simulink model "MATE_SynchronousMachine"  (R2024b)
settings: Solver=FixedStepDiscrete  StartTime=0.0  StopTime=6  FixedStep=Ts  RelTol=1e-4  EnableMultiTasking=on
PostLoadFcn:
  | Ts=25e-6;offset=4;
InitFcn:
  | Ts=25e-6;offset=4;
undefined symbols (not defined in the file): DiscIntNeverNeededParam, MATE, Phase, Rsnu, Single
libraries: fl_lib x79, nesl_utility x53, ee_lib x16, simetran x5, powerlib_extras x3, simulink_extras x2, simulink x2
(part 1 of 5)
settings Model: ARTEMISmethode_block_infos=$$__separator__$$  Creator=by2815  LastModifiedBy=CD8435
settings SolverCC: AlgebraicLoopSolver=TrustRegion
settings DataIOCC: SaveFormat=Structure  SignalLoggingSaveFormat=ModelDataLogs  SaveOutput=off  SignalLogging=off  SaveTime=off  ReturnWorkspaceOutputs=off  SignalLoggingName=sigsOut
settings OptimizationCC: ExpressionDepthLimit=2147483647  InitFltsAndDblsToZero=on  LifeSpan=inf
settings DebuggingCC: SaveWithParameterizedLinksMsg=none  UnderspecifiedInitializationDetection=Classic  MergeDetectMultiDrivingBlocksExec=none  SignalResolutionControl=TryResolveAllWithWarning  MultiTaskDSMMsg=warning  MultiTaskCondExecSysMsg=none  FcnCallInpInsideContextMsg=warning  AllowSymbolicDim=off  StateNameClashWarn=warning  NonBusSignalsTreatedAsBus=error  SFUnexpectedBacktrackingDiag=warning  SFNoUnconditionalDefaultTransitionDiag=warning  SFExecutionAtInitializationDiag=none  ArithmeticOperatorsInVariantConditions=warning
settings HardwareCC: ProdBitPerPointer=32  ProdBitPerSizeT=32  ProdBitPerPtrDiffT=32  ProdLargestAtomicFloat=None  ProdIntDivRoundTo=Undefined  ProdEndianess=Unspecified  ProdWordSize=32  ProdHWDeviceType=32-bit Generic  TargetUnknown=on
settings ModelReferenceCC: EnableRefExpFcnMdlSchedulingChecks=on  PropagateSignalLabelsOutOfModel=off
settings SFSimCC: SimUseLocalCustomCode=off  CustomCodeUndefinedFunction=UseInterfaceOnly
settings RTWCC: RTWUseLocalCustomCode=off  GPUComputeCapability=3.5
settings CodeAppCC: StateflowObjectComments=on
settings GRTTargetCC: TargetFcnLib=ansi_tfl_tmw.mat  TargetLangStandard=C89/C90 (ANSI)  CombineOutputUpdateFcns=off  GRTInterface=on
settings ConfigComp: CovMetricSettings=dw  CovSaveCumulativeToWorkspaceVar=on  CovSaveSingleToWorkspaceVar=on  CovExternalEMLEnable=off
settings SimscapeCC: SimscapeNormalizeSystem=off

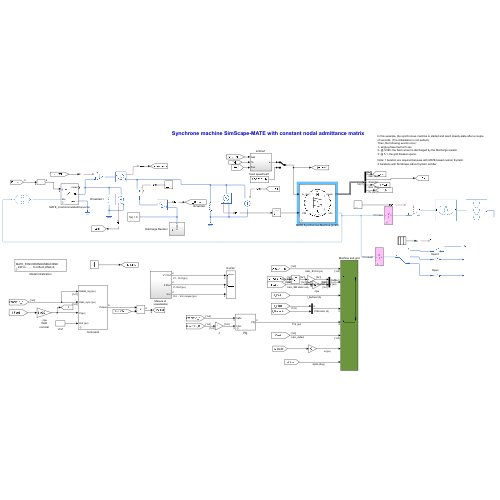
[thumbnail: Simulink's stored preview of the top-level diagram]
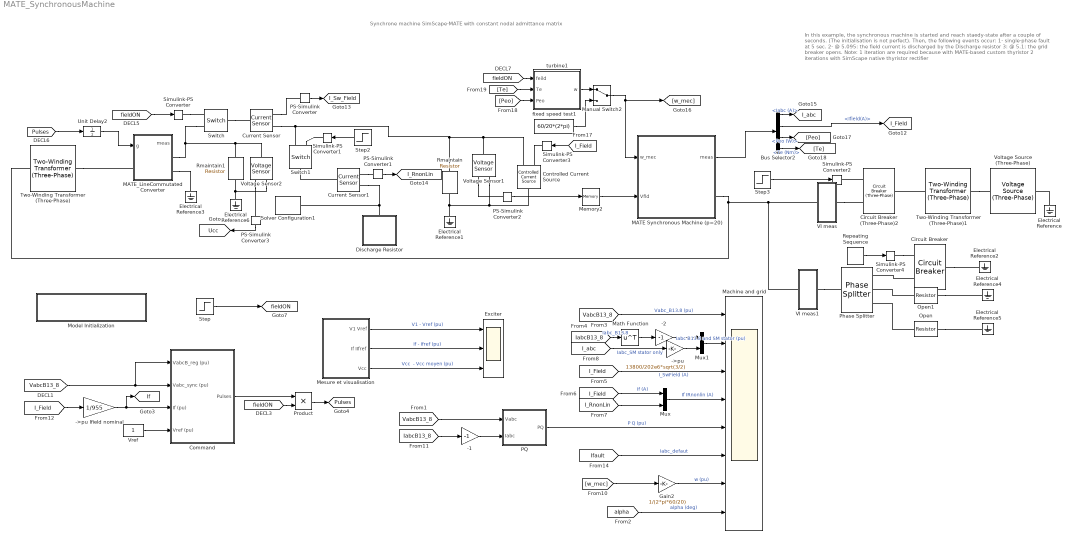
== system MATE_SynchronousMachine ==
  note: In this example, the synchronous machine is started and reach staedy-state after a couple of seconds. (The initialisation is not perfect).
      | Then, the following events occur:
      | 1- single-phase fault at 5 sec.
      | 2- @ 5.095: the field current is discharged by the Discharge resistor
      | 3: @ 5.1: the grid breaker opens.
      |
      | Note: 1 iteration are required because with MATE-based custom thyristor
      | 2 iterations with SimScape native thyristor rectifier
  note: Synchrone machine SimScape-MATE with constant nodal admittance matrix
  -1 : Gain  Gain=-1
  -2 : Gain  Gain=-1
  ->pu : Gain  Gain=13800/202e6*sqrt(3/2)
  ->pu Ifield nominal : Gain  Gain=1/955
  Bus Selector2 : BusSelector  OutputSignals=Iabc (A),Ifield(A),Peo (W),Te (Nm)
  Circuit Breaker : ee_lib/Switches & Breakers/Circuit Breaker  R_closed=0.01 Ohm  G_open=1e-6 1/Ohm  threshold=0.5 V  breaker_behavior=ee.enum.switches.breakerBehavior.zeroCrossingEnable
      settings: InternalSimscapePortConfiguration="{\"Bottom\":[],\"Left\":[{\"id\":\"vT\",\"label\":\"vT\",\"type\":\"input\"},{\"id\":\"p1\",\"label\":\"\",\"type\":\"foundation.electrical.electrical\"}],\"Right\":[{\"id\":\"p2\",\"label\":\"\",\"type\":\"foundation.electrical.electrical\"}],\"Top\":[]}"
  Circuit Breaker (Three-Phase)2 : ee_lib/Switches & Breakers/Circuit Breaker (Three-Phase)  R_closed=0.01 Ohm  G_open=1e-6 1/Ohm  threshold=0.5 V  breaker_behavior=ee.enum.switches.breakerBehavior.zeroCrossingEnable
      settings: InternalSimscapePortConfiguration="{\"Bottom\":[],\"Left\":[{\"id\":\"vT\",\"label\":\"vT\",\"type\":\"input\"},{\"id\":\"N1\",\"label\":\"~1\",\"type\":\"foundation.electrical.three_phase\"}],\"Right\":[{\"id\":\"N2\",\"label\":\"~2\",\"type\":\"foundation.electrical.three_phase\"}],\"Top\":[]}"
  Command : Subsystem  mask{ModOp=Automatique (regulation de tension), Vref=1.0, Iref_man=1.0, K_V=[ 20 300  ], K_I=[ 400  1000 ], Ts=Ts}
      mask prompts: ModOp "Mode d'operation"; Vref "Consigne de tension (pu)"; Iref_man "Consigne de courant (pu)"; K_V "Gain du regulateur de tension [ Kp  Ki ]"; K_I "Gain du regulateur de courant: [ Kp  Ki ]"; Ts "Pas de calcul"
      mask init:
      | Kp_V=K_V(1); Ki_V=K_V(2);
      | Kp_I=K_I(1); Ki_I=K_I(2);
      | if ModOp==1
      |     Auto=1;
      | else
      |     Auto=0;
      | end
      mask TypeOptions ModOp: Automatique (regulation de tension) | Manuel (regulation de courant)
  Controlled Current Source : fl_lib/Electrical/Electrical Sources/Controlled Current Source
  Current Sensor : fl_lib/Electrical/Electrical Sensors/Current Sensor
  Current Sensor1 : fl_lib/Electrical/Electrical Sensors/Current Sensor
  Discharge Resistor : Subsystem
  Electrical Reference{,1..6} (7 alike) : fl_lib/Electrical/Electrical Elements/Electrical Reference
  Exciter : Scope  NumInputPorts=3
  Gain2 : Gain  Gain=1/(2*pi*60/20)
  MATE Synchronous Machine (p=20) : Subsystem  mask(MATE Synchronous Machine (Fixed Admittance)){NominalParameters=[ 202e6  13800   60   955 ], Rtype=Salient (5ft order model), Stator=[ 2.9069E-03  3.0892E-04  3.2164E-03 9.7153E-04 0.0], Field=[ 5.9013E-04*0.128/0.08381   3.0712E-04], Dampers1=[ 1.1900E-02  4.9076E-04   2.0081E-02  1.0365E-03  2.0081E-02  1.0365E-03], PolePairs=20, InitialConditions=-95, InitCurrents=[ 1180 9560 9560 9650 [0 -120 120]-95], Ts=Ts, Parameter19=|, sat=off, DiffSat=off, SatVt=[0 0.7 1 1.4], SatIfd=[0 0.5 1 2], plotsat=off, R0=500, X0=0.11643, nsnf_readonly=0.083912, Parameter18=|}
      mask Parameter19=|
      | Saturation: Saturation is used if selected
      |
      | Open stator saturation curve: field current data in per unit of nominal field current
      | Open stator saturation curve: phase-phase RMS terminal voltage in per unit of nominal voltage
      | Plot saturation curves
      | Zero sequence machine reactance (Ohms): grounding impedance internally connected to the stator Y neutral.
      | Neutral grounding resistance (Ohms): grounding resistance (in series with the impedance) internally connected to the stator Y neutral.
      mask Parameter18=|
      | The stator-to-field coil winding turn ratio (Ns_to_Nf) is found using the following formula:
      |
      | Ns_on_Nf=Lmd*I_fn*(2*pi*f_base)/Vbase
      | where Lmd (d-axis mutual inductance), I_fn (nominal field current), f_base (nominal electric frequency) and Vbase (open-stator machine nominal line-line RMS voltage).
      mask prompts: NominalParameters "Nominal power, voltage, frequency, field current  [ Pn(VA) Vn(Vrms) fn(Hz) ifn(A) ]:"; Rtype "Rotor type"; Stator "Stator  [ Rs(ohm), Ll, Lmd, Lmq(H), Lcanay(H) ]:"; Field "Field  [ Rf'(ohm)  Llfd'(H) ]:"; Dampers1 "Dampers   [ Rkd',Llkd'  Rkq1',Llkq1'  Rkq2' Llkq2' ] (R=ohm,L=H): (Rk2 Lfk2 values not used for salient type machine)"; PolePairs "Pole pairs:"; InitialConditions "Initial rotor angle (deg):"; InitCurrents "Initial currents  Ifd (A) Ia Ib Ic (A) (amplitude)  Ia Ib Ic (deg)(angle )"; Ts "Sample Time (s)"; Parameter19 "text1"; sat "Saturation"; DiffSat "Differential saturation (not available)"; SatVt "Open stator saturation curve: phase-phase RMS voltage (pu of nominal voltage)"; SatIfd "Open stator saturation curve: field current (pu of nominal field current)"; plotsat "Plot saturation curves"; R0 "Neutral grounding resistance (Ohms)"; X0 "Zero sequence machine reactance (Ohms)"; nsnf_readonly "Computed Stator/Field turn ratio (read-only)"; Parameter18 "text2"
      mask help:
      | Implements a 3-phase synchronous machine modelled in the dq rotor reference frame for use with SimScape
      | The model uses a fixed admittance matrix method and is well designed for real-time simulation.
      |
      | The model is 6th order for the round rotor type and 5th order for the salient rotor type (Rk2 Llk2 are internally set to inf in this case).Stator windings are connected in wye to an internal neutral point to which an internal impedance to ground can be selected by the user.
      | If selected, saturation occured in both d- and q- axis, using total flux, for the round and salient rotor type.
      |
      |
      | Parameters: (all values are in SI units)
      |
      | Nominal power, voltage, frequency, field current  [ Pn(VA) Vn(Vrms) fn(Hz) ifn(A) ]: nominal values for total power, line-line RMS voltage, frequency and field current
      | Rotor type: Salient (5ft order model)/Round (6th order model)
      | Stator  [ Rs(ohm), Ll, Lmd, Lmq(H) Lcanay(H)]: Stator resistance and leakage inductance, magnetization inductance for d-q axes.The 5th element is the Canay inductance, which can set to 0 if unknown. The Canay inductance applies a correction for the coupling between damper and field windgins in the d-axis.
      | Field  [ Rf'(ohm)  Llfd'(H) ]: Field resistance and leakage inductance (seen from the stator)
      | Dampers   [ Rkd',Llkd'  Rkq1',Llkq1'  Rkq2' Llkq2' ] (R=ohm,L=H): (Rk2 Lfk2 values not used for salient type machine):
      | Pole pairs: number of pair of poles
      | Initial rotor angle  (deg): initial rotor angle in degree.
      | Initial currents  Ifd Ia Ib Ic (A) (amplitude)  Ia Ib Ic (deg)(angle )
      | Sample Time (s) : Sample time of the model in seconds
      mask init:
      | block = gcb;
      | ddst='on';  % delay spedd term always in Fixed Admittance model
      | 
      | 
      | 
      | Lmd=Stator(3);
      | Lmq=Stator(4);
      | Lls=Stator(2);
      | Lcanay=0;
      | if length(Stator)==5
      |     Lcanay=Stator(5);
      | end
      |     
      | Ld=Lmd+Lls;
      | Lq=Lmq+Lls;
      | Rs=Stator(1);
      | Rf=Field(1);
      | Llf=Field(2);
      | Lf=Lmd+Llf;
      | Rkd=Dampers1(1);
      | Llkd=Dampers1(2);
      | Lkd=Lmd+Llkd;
      | Rkq=Dampers1(3);
      | Llkq=Dampers1(4);
      | Lkq=Lmq+Llkq;
      | Rkq2=Dampers1(5);
      | Llkq2=Dampers1(6);
      | Lkq2=Lmq+Llkq2;
      | 
      | 
      | 
      | 
      | Lad =1/(1/Lmd+1/Lls+1/Llkd+1/Llf);
      | Laq =1/(1/Lmq+1/Lls+1/Llkq+1/Llkq2);
      | 
      | pp=PolePairs;
      | Sbase=NominalParameters(1);
      | Vbase=NominalParameters(2); % *sqrt(2/3);
      | wbase=NominalParameters(3)*2*pi;
      | Zbase=Vbase*Vbase/Sbase;
      | Ibase=Vbase/Zbase;
      | Lbase=Zbase/wbase;
      | %PhiBase=Lbase*Ibase;
      | PhiBase=Vbase*sqrt(2/3)/wbase;  % real flux base. ref: Gilbert Sybille IREQ
      | I_field_nominal=NominalParameters(4);
      | Ifd_base=I_field_nominal*Lmd/Lbase;
      | 
      | Ns_on_Nf_noLmd=I_field_nominal*wbase/Vbase;
      | Ns_on_Nf=Lmd*I_field_nominal*wbase/Vbase;  % stator/field turn ratio
      | set_param(block,'nsnf_readonly',num2str(Ns_on_Nf));
      | 
      | theta_0=(InitialConditions(1)-90)/180*pi;  % orthonormal Park transform has a 90 deg shift with the conventional SPS Park transform
      | 
      | S=[cos(theta_0) sin(theta_0);-sin(theta_0) cos(theta_0)];
      | 
      | T=S*sqrt(2/3)*[1 -0.5 -0.5;0 sqrt(3)/2 -sqrt(3)/2];
      | 
      | 
      | 
      | % Conversion of initial current phasors to instantaneous values
      | [iau,iao] = pol2cart((InitCurrents(5))*pi/180,InitCurrents(2));
      | [ibu,ibo] = pol2cart((InitCurrents(6))*pi/180,InitCurrents(3));
      | [icu,ico] = pol2cart((InitCurrents(7))*pi/180,InitCurrents(4));
      | 
      | idq=T*(-1)*[iao;ibo;ico];  %-1 here, don't know why exactly...
      | 
      | 
      | 
      | if isequal(get_param(block, 'Rtype'),'Salient (5ft order model)')
      |     nb_row=5;
      |     nb_row3=2;
      |     list_row=[2 5];
      |     Rkq2=0;
      |     Llkq2=inf;
      |     Lkq2=inf;
      |     L0=[Ld 0 Lmd Lmd 0 ; 0 Lq 0 0  Lmq ; Lmd 0 Lf Lmd 0 ; Lmd 0 Lmd Lkd 0  ; 0 Lmq 0 0 Lkq ];
      |     flux_0=L0*[idq;InitCurrents(1)/Ns_on_Nf;0;0]; % initial conditions
      |     dsatOnly=1;  % d-axis saturation only
      |  
      | 
      | MD=(Lmd+Lmq)/2;
      | LD=MD+Lls;
      | LQ=LD;
      | RD=Rs*eye(3);
      | 
      | LDD=[LD MD MD;MD LD MD;MD MD LD];
      | LQQ=[LD MD ;MD LD]; 
      | invD=inv(LDD);
      | RinvD=RD*invD;
      | invQ=[invD(1,1) invD(2,1); invD(2,1) invD(1,1)];
      | 
      | 
      | Yd=invD*inv(eye(3)+Ts/2*RD*invD);
      | Yd22=[Yd(1,1) Yd(1,2); Yd(2,1) Yd(2,2)];
      | 
      | RQ2=2/Ts*inv(Yd22)*(invQ-Yd22)*inv(invQ);
      | 
      | Yq=invQ*inv(eye(2)+Ts/2*RQ2*invQ);
      | 
      | LDx=invD(1,1);
      | MDx=invD(2,1);
      | 
      | RQ=RQ2;
      | 
      | invLavg=[LDx 0 MDx MDx 0; 0 LDx 0 0 MDx ;MDx 0 LDx MDx 0 ;MDx 0 MDx LDx 0 ;0 MDx 0 0 LDx];
      | 
      | Ravg=[Rs 0 0 0 0; 0 RQ(1,1) 0 0 RQ(1,2) ;0 0 Rs 0 0 ;0 0 0 Rs 0 ;0 RQ(1,2) 0 0 RQ(1,1)];
      | RinvLavg=Ravg*invLavg;
      | aaa=RD*invD;
      | bbb=RQ*invQ;
      | RLDx=aaa(1,1);RMDx=aaa(2,1);
      | RLQx=bbb(1,1);RMQx=bbb(2,1);
      | RinvLavg=[RLDx 0 RMDx RMDx 0; 0 RLQx 0 0 RMQx ;RMDx 0 RLDx RMDx 0 ;RMDx 0 RMDx RLDx 0 ;0 RMQx 0 0 RLQx];
      | 
      | 
      | Lmat=[Ld 0 Lmd Lmd 0 ; 0 Lq 0 0  Lmq ; Lmd 0 Lf+Lcanay Lmd+Lcanay 0 ; Lmd 0 Lmd+Lcanay Lkd+Lcanay 0  ; 0 Lmq 0 0 Lkq ];
      | invLmat=inv(Lmat);
      | Rmat=[Rs 0 0 0 0 ; 0 Rs 0 0 0 ; 0 0 Rf  0 0 ; 0 0 0 Rkd 0 ; 0 0 0 0  Rkq ];
      | moinsRmatinvLmat=-Rmat*invLmat;
      | 
      | Ydq=[Yd(1,1) 0 Yd(1,2) Yd(1,3) 0; 0 Yq(1,1) 0 0 Yq(1,2); Yd(2,1) 0 Yd(2,2) Yd(2,3) 0; Yd(3,1) 0 Yd(3,2) Yd(3,3) 0; 0 Yq(2,1) 0 0 Yq(2,2)];
      | 
      | %refine T for the rest...
      | T=[1 0;0 1]*sqrt(2/3)*[1 -0.5 -0.5;0 sqrt(3)/2 -sqrt(3)/2];
      | T=cat(2,T,[0 0]');
      | T=cat(1,T,[0 0 0 1; 0 0 0 0;0 0 0 0]);
      | 
      | 
      | Y44=Ts/2*T'*Ydq*T;
      | Y=Y44(1:3,1:3);
      | 
      | 
      | else
      |     nb_row=6;
      |     nb_row3=3;
      |     list_row=[2 5 6];
      |     L0=[Ld 0 Lmd Lmd 0 0; 0 Lq 0 0  Lmq Lmq; Lmd 0 Lf Lmd 0 0; Lmd 0 Lmd Lkd 0 0 ; 0 Lmq 0 0 Lkq Lmq;0 Lmq 0 0 Lmq Lkq2];
      |     flux_0=L0*[idq;InitCurrents(1)/Ns_on_Nf;0;0;0]; % initial conditions
      |     dsatOnly=0;
      |     Ldq2=(Ld+Lq+Lf+Lkd+Lkq+Lkq2)/6;
      |     Ravg=(Rs+Rs+Rf+Rkd+Rkq+Rkq2)/6;
      |     Lmdq2=(1*Lmd+1*Lmq)/2;
      |     Lavg=[Ldq2 0 Lmdq2 Lmdq2 0 0; 0 Ldq2 0 0 Lmdq2 Lmdq2;Lmdq2 0 Ldq2 Lmdq2 0 0;Lmdq2 0 Lmdq2 Ldq2 0 0;0 Lmdq2 0 0 Ldq2 Lmdq2; 0 Lmdq2 0 0 Lmdq2 Ldq2];
      |     invLavg=inv(Lavg);
      |     
      |     RinvLavg=Ravg*invLavg;
      | Lmat=[Ld 0 Lmd Lmd 0 0; 0 Lq 0 0  Lmq Lmq; Lmd 0 Lf+Lcanay Lmd+Lcanay 0 0; Lmd 0 Lmd+Lcanay Lkd+Lcanay 0 0 ; 0 Lmq 0 0 Lkq Lmq;0 Lmq 0 0 Lmq Lkq2];
      | Rmat=[Rs 0 0 0 0 0; 0 Rs 0 0 0 0; 0 0 Rf  0 0 0; 0 0 0 Rkd 0 0; 0 0 0 0  Rkq 0; 0 0 0 0 0 Rkq2];
      | invLmat=inv(Lmat);
      | moinsRmatinvLmat=-Rmat*invLmat;
      | 
      | % Yd=invD*inv(eye(3)+Ts/2*RD*invD);
      | % Yd22=[Yd(1,1) Yd(1,2); Yd(2,1) Yd(2,2)];
      | % 
      | % RQ2=2/Ts*inv(Yd22)*(invQ-Yd22)*inv(invQ);
      | % 
      | % Yq=invQ*inv(eye(2)+Ts/2*RQ2*invQ);
      | 
      | %refine T for the rest... one more row of 0 here...
      | T=[1 0;0 1]*sqrt(2/3)*[1 -0.5 -0.5;0 sqrt(3)/2 -sqrt(3)/2];
      | T=cat(2,T,[0 0]');
      | T=cat(1,T,[0 0 0 1; 0 0 0 0;0 0 0 0; 0 0 0 0]);
      | 
      | %Ts/2*Ravg*invLavg
      | Ydq=invLavg*inv(eye(6)+Ts/2*Ravg*invLavg);
      | Y44=Ts/2*T'*Ydq*T;
      | Y=Y44(1:3,1:3);
      | 
      | 
      | end
      | 
      | % zero-sequence admittance
      | T0=[1 1 1]*sqrt(1/3);
      | invL0=wbase/X0;
      | Ac0=-(Rs+R0)*invL0;
      | Y0=Ts/2*T0'*invL0*inv(1-Ts/2*Ac0)*T0;
      | 
      | % setting external resistances 
      | ResistanceM=zeros(3,3);
      | Ytot=Y+Y0;
      | ResistanceM(1,1)= 1/sum(Ytot(1,:));
      | ResistanceM(2,2)= 1/sum(Ytot(2,:));
      | ResistanceM(3,3)= 1/sum(Ytot(3,:));
      | ResistanceM(1,2)=-1/(Ytot(1,2));
      | ResistanceM(1,3)=-1/(Ytot(1,3));
      | ResistanceM(2,1)=-1/(Ytot(2,1));
      | ResistanceM(2,3)=-1/(Ytot(2,3));
      | ResistanceM(3,1)=-1/(Ytot(3,1));
      | ResistanceM(3,2)=-1/(Ytot(3,2));
      | 
      | 
      | 
      | 
      | 
      | Ifd=str2num(get_param(block,'SatIfd'));
      | Vt=str2num(get_param(block,'SatVt'));
      | Ifd=Ifd*I_field_nominal;   % modif 17 mai 2017: Vt=f(Ifd) en pu
      | Vt=Vt*Vbase;
      | if sat==0
      |     set_param(block,'DiffSat','off');
      | end
      | 
      | if sat==1
      |     %Vbase=NominalParameters(2);
      |     %wbase=NominalParameters(3)*2*pi;
      |     %PhiBase=Vbase*sqrt(2/3)/wbase;  % real flux base ref: Gilbert Sybille IREQ
      |     %I_field_nominal=NominalParameters(4);
      |     %Ns_on_Nf=Lmd*I_field_nominal*wbase/Vbase;  % stator/field turn
      |     
      |     if length(Ifd)~=length(Vt)
      |         error('Saturation field current and voltage must have the same length');
      |     end
      |     if length(Ifd)<2
      |         error('Saturation field current and voltage must have a minimum length of 2, including the (0,0) point');
      |     end
      |     if Ifd(1)~=0 | Vt(1)~=0
      |         error('Saturation field current and voltage must include the (0,0) point');
      |     end
      |     
      |     %Vt=Lmd*I_field_nominal*wbase/Ns_on_Nf;
      |     %Lmd_sat=Vt*Ns_on_Nf/Ifd/wbase;
      |     % find nominal magnetizing inductance from the saturation curve
      |     for i=2:length(Ifd)
      |         if Ifd(i)>I_field_nominal
      |             break
      |         end
      |     end
      |     pente=(Vt(i)-Vt(i-1))/(Ifd(i)-Ifd(i-1));
      |     Vtnom_sat=Vt(i-1)+(I_field_nominal-Ifd(i-1))*pente;
      |     Lnom=Vtnom_sat/I_field_nominal;  % slope at nominal field current
      |     table_saturation_factor=(Vt(2:end)./Ifd(2:end))/Lnom;
      |     table_saturation_factor=[table_saturation_factor(1) table_saturation_factor];
      |     % careful with point 0,0...
      |     %table_flux_input=Vt*sqrt(2/3)/wbase;
      |     table_flux_input=Vt/wbase;  % the sqrt(2/3) factor is not required here
      |     
      | else
      |     table_saturation_factor=[1 1 1];
      |     table_flux_input=[0 1 2];
      |     
      | end
      | 
      | Vx=Vt'/wbase;
      | b=Ifd'/Ns_on_Nf;
      | 
      | if DiffSat==1
      |     if length(Ifd)~=4
      |         error('When using differential saturation, saturation field current and voltage must be a vector of 4 of length');
      |     end
      |     
      |     
      |     %Lmd=(Vf/wbase)/(Ifd/Ns_on_Nf)
      |     % fitting exact with 4 points
      |     % y=a+b*x+c*x^2+d*x^3    x is voltage/wbase  b is Ifd/Ns_on_Nf
      |     % so we are looking for a function of Vstator or flux here
      |     % b=Vt'/wbase;
      |     % Ix=Ifd/Ns_on_Nf;
      |     % A(:,1)=[1 1 1 1]';
      |     % A(:,2)=Ix';
      |     % A(:,3)=(Ix.*Ix)';
      |     % A(:,4)=(Ix.*Ix.*Ix)';
      |     
      |     A(:,1)=[1 1 1 1]';
      |     A(:,2)=Vx';
      |     A(:,3)=(Vx.*Vx)';
      |     A(:,4)=(Vx.*Vx.*Vx)';
      |     
      |     w=inv(A)*b;
      | else
      |     w=[1;1;1;1];
      |     
      | end
      | 
      | 
      | if plotsat
      |     figure
      |     if DiffSat==1
      |         x=0:Vx(end)/20:Vx(end);
      |         y=w(1)+x.*w(2)+x.*x.*w(3)+x.*x.*x.*w(4);  %fitted curve i=f(v) car on veut une fonction de v (ou flux)
      |         plot(b*Ns_on_Nf,Vx*wbase,'*b');
      |         hold on
      |         plot(y*Ns_on_Nf,x*wbase,'r');  % put current on x-axis
      |         xlabel('Field current (A)');
      |         ylabel('Open stator terminal voltage (V)');
      |         
      |         slopee=w(2)+2*w(3).*Vx+3*w(4).*Vx.*Vx;
      |         offsett=w(1)-w(3).*Vx.*Vx-2*w(4).*Vx.*Vx.*Vx;
      |         slope_inv=1./slopee;
      |         offset_inv=-offsett./slopee;  % pente et offset de la courbe v=f(i)
      |         ifdvec=0:b(end)/20:b(end);
      |         for ii=2:length(slope_inv)
      |             vv=offset_inv(ii)+slope_inv(ii).*ifdvec;
      |             plot(ifdvec*Ns_on_Nf,vv*wbase,'g');
      |         end
      |         legend('user data point','fitted curve','linear approx at user points','Location','NorthWest')
      |         
      |         
      |         hold off
      |         
      |     else
      |         plot(b*Ns_on_Nf,Vx*wbase,'*-b');
      |         hold
      |         plot([I_field_nominal I_field_nominal],[0 Vbase],'-r');
      |         plot([0 I_field_nominal],[Vbase Vbase],'-r');
      |         xlabel('Field current (A)');
      |         ylabel('Open stator terminal voltage (V)');
      |         title ('red line indicate nominal point');
      |         hold off
      |     end   
      | end
      |     set_param(block,'plotsat', 'off');
      | 
      | 
      | 
      | 
      | 
      | % no more goto-from in this fixed admittance model
      | %added by Opal-RT
      | % tagg=get_param(block,'taggg');
      | % set_param([gcb '/FromV'],'GotoTag',['ssn_ext_sys_from_V_' tagg]);
      | % set_param([gcb '/GotoHist'],'GotoTag',['ssn_ext_sys_goto_Hist_' tagg]);
      | % set_param([gcb '/GotoY'],'GotoTag',['ssn_ext_sys_goto_Y_' tagg]);
      | 
      | %set_param([gcb '/SSN-SM'],'taggg',tagg);
      | 
      | %NomParams=get_param(block,'NominalParameters');
      | %NomParams=getSPSmaskvalues(block,{'NominalParameters'});
      | 
      | %Ifn=NomParams(4);
      | % icon plot
      | 
      | 
      | % set model speed term routing
      | if isequal(ddst, 'on')
      |     o1=0;
      |     o2=1:(nb_row+4);
      | 
      | else
      |     o1=1;
      |     o2=1:4;
      | 
      | end
      mask TypeOptions Rtype: Salient (5ft order model) | Round (6th order model)
      mask Callback sat:
      | block = gcb;
      | sattt=get_param(block,'sat');
      | 
      | % hide saturation option if saturation not selected
      | visib=get_param(block,'MaskVisibilities');
      | if isequal(sattt,'on')
      |     visib{12}='on';visib{13}='on';visib{14}='on';visib{15}='on';
      | else
      |     visib{12}='off';visib{13}='off';visib{14}='off';visib{15}='off';
      | end
      | visib{11}='on';
      | set_param(block,'MaskVisibilities',visib);
      mask DialogControl ParameterTabVar0 Prompt: Parameters
      mask DialogControl Container5 Prompt: Saturation and zero sequence
      mask DialogControl ParameterTabVar01 Prompt: More Info
  MATE_LineCommutatedConverter : Subsystem  AncestorBlock=simetran/MATE_LineCommutatedConverter  mask(MATE 3-phase Diode/Thyristor Rectifier){umate=on, sd=Thyristors, ron=1e-2, roff=1e5, vf=1, rcs=on, rsnu=100, csnu=2e-6, ts=Ts}
      mask prompts: umate "Use MATE aggregated model"; sd "Switching Device"; ron "Ron (Ohms)"; roff "Roff (Ohms)"; vf "Forward voltage drop (V)"; rcs "RC snubber (otherwise only R)"; rsnu "Snubber resistance (Ohms)"; csnu "Snubber capacitance (Ohms)"; ts "Sample time (s)"
      mask init:
      | bloc=gcb;
      | 
      | if isequal(get_param(bloc,'rcs'), 'on')
      |     RCsnubber=1;
      | else
      |     RCsnubber=0;
      | end
      | bloc=gcb;
      | um=get_param(bloc,'umate');
      | if isequal (um,'on')
      | [MATE,MATERT]=Compute_6_pulse_thy_Fnc(bloc, 4, rsnu,csnu, RCsnubber,ron,ts,1,vf);
      | end
      mask Callback umate:
      | bloc=gcb;
      | um=get_param(bloc,'umate');
      | if isequal (um,'on')
      |     set_param([bloc '/MATE_AGGREG'], 'Commented', 'off');
      |     set_param([bloc '/MATEPREP'], 'Commented', 'on');
      | else
      |     set_param([bloc '/MATE_AGGREG'], 'Commented', 'on');
      |     set_param([bloc '/MATEPREP'], 'Commented', 'off');
      | end
      mask TypeOptions sd: Diodes | Thyristors
  Machine and grid : Scope  NumInputPorts=8
  Manual Switch2 : ManualSwitch
  Math Function : Math  Operator=transpose
  Memory2 : Memory
  Mesure et visualisation : Subsystem
  Model Initialization : Subsystem  AncestorBlock=artemis/Tools /Misc/Model Initialization  mask(Model Functions){InitFcnX=Ts=25e-6;offset=4;, prel=off, posl=on, inif=on, strf=off}
      mask prompts: InitFcnX "Initialisation"; prel "Preload Function"; posl "PostLoad Function"; inif "InitFcn"; strf "StartFcn"
      mask init:
      | currentBlock = gcb;
      | root = bdroot(currentBlock);
      | 
      | if ~strcmp(get_param(root,'BlockDiagramType'),'library')
      |     if prel==1
      |         set_param(root, 'PreLoadFcn', InitFcnX);
      |     else
      |         set_param(root, 'PreLoadFcn', '');
      |     end
      |     if inif==1
      |         set_param(root, 'InitFcn', InitFcnX);
      |     else
      |         set_param(root, 'InitFcn', '');
      |     end
      |     if strf==1
      |         set_param(root, 'StartFcn', InitFcnX);
      |     else
      |         set_param(root, 'StartFcn', '');
      |     end
      |     if posl==1
      |         set_param(root, 'PostLoadFcn', InitFcnX);
      |     else
      |         set_param(root, 'PostLoadFcn', '');
      |     end
      | end
      | 
      | pos = get_param(currentBlock, 'Position');
      | width = pos(3) - pos(1); height = pos(4) - pos(2);
      | txt = [ upper(root) '\n' '- InitFcn. . . . . '  get_param(root, 'InitFcn') ];
      settings: CopyFcn=set_param(gcb,'LinkStatus','inactive')
      mask Display: text(5, height*0.5, txt, 'horizontalAlignment', 'left', 'verticalAlignment', 'middle') ;
  Mux : Mux  Inputs=2
  Mux1 : Mux  Inputs=2
  Open : fl_lib/Electrical/Electrical Elements/Resistor  R=1e8 Ohm  i_specify=off  i_priority=None  i=0 A  i_nominal_specify=off  i_nominal_value=1  i_nominal_unit=A  v_specify=off  v_priority=None  v=0 V  v_nominal_specify=off  v_nominal_value=1  v_nominal_unit=V
  Open1 : fl_lib/Electrical/Electrical Elements/Resistor  R=1e8 Ohm  i_specify=off  i_priority=None  i=0 A  i_nominal_specify=off  i_nominal_value=1  i_nominal_unit=A  v_specify=off  v_priority=None  v=0 V  v_nominal_specify=off  v_nominal_value=1  v_nominal_unit=V
  PQ : Subsystem  mask(3-phase instantaneous active and reactive power){}
      mask init:
      | power_initmask();
      mask Display: disp('')
  PS-Simulink Converter{,1..3} (4 alike) : nesl_utility/PS-Simulink Converter  PhysicalDomain=network_engine_domain  SubClassName=ps_output  LeftPortType=input  RightPortType=output  PseudoPeriodic=off  Frequencies=[]  VectorFormat=inherit  Unit=inherit  AffineConversion=off
  Phase Splitter : ee_lib/Connectors & References/Phase Splitter
  Product : Product
  Repeating Sequence : simulink/Sources/Repeating Sequence  rep_seq_t="[0   [1-Ts 1  1.15-Ts 1.15]+offset  100]"  rep_seq_y="[1     1    0      0        1                1]"
  Rmaintain : fl_lib/Electrical/Electrical Elements/Resistor  R=5000 Ohm  i_specify=off  i_priority=None  i=0 A  i_nominal_specify=off  i_nominal_value=1  i_nominal_unit=A  v_specify=off  v_priority=None  v=0 V  v_nominal_specify=off  v_nominal_value=1  v_nominal_unit=V
  Rmaintain1 : fl_lib/Electrical/Electrical Elements/Resistor  R=50000 Ohm  i_specify=off  i_priority=None  i=0 A  i_nominal_specify=off  i_nominal_value=1  i_nominal_unit=A  v_specify=off  v_priority=None  v=0 V  v_nominal_specify=off  v_nominal_value=1  v_nominal_unit=V
  Simulink-PS Converter{,1..4} (5 alike) : nesl_utility/Simulink-PS Converter  PhysicalDomain=network_engine_domain  SubClassName=ps_input  LeftPortType=input  RightPortType=output  PseudoPeriodic=off  Frequencies=[]  NoiseDistribution=none  NoiseParameters=[]  Unit=1  AffineConversion=off  FilteringAndDerivatives=provide  SimscapeFilterOrder=1  InputFilterTimeConstant=0.001  UdotUserProvided=0
  Solver Configuration1 : nesl_utility/Solver Configuration  PhysicalDomain=network_engine_domain  SubClassName=solver  LeftPortType=input  RightPortType=generic  Tones=[]  Harmonics=[]  SimulateNoise=off  Profile=off  UseLocalSampling=off  EnableSwitchedLinearOptims=on  FrequencyDomain=off  UseCCode=off  RelTol=0.001  AbsTol=1e-06  MinStep=1e-09  ToWorkspace=off  RevertToSquareIcSolve=off  NumHomotopyIterations=100  PhasorMode=off  PhasorModeNumHarmonics=1  ConsistencySolver=NEWTON_FTOL  IndexReductionMethod=DerivativeReplacement  DoDC=off  ResidualTolerance=0.001  ConsistencyTolSource=GLOBAL  ConsistencyAbsTol=0.001  ConsistencyRelTol=0.001  ConsistencyTolFactor=0.001  UseLocalSolver=on  LocalSolverChoice=NE_BACKWARD_EULER_ADVANCER  ResolveIndetEquations=off  FunctionEvalNumThread=1  LocalSolverSampleTime=Ts  DoFixedCost=on  MaxNonlinIter=1  MaxModeIter=2  ComputeImpulses=off  ImpulseIterations=2  LinearAlgebra=Sparse  LinearAlgebraNumThread=0  EquationFormulation=NE_TIME_EF  DelaysMemoryBudget=1024  AutomaticFiltering=off  FilteringTimeConstant=0.001  PartitionStorageMethod=AS_NEEDED  PartitionMemoryBudget=1024  PartitionMethod=ROBUST  MultibodyUseLocalSolver=off  MultibodyLocalSolverChoice=ODE1  MultibodyLocalSolverSampleTime=0.001
  Step : Step  Time=1.1+offset  Before=1  After=0  SampleTime=0
  Step2 : Step  Time=1.095+offset  SampleTime=0
  Step3 : Step  Time="[ 1.1+offset  ]"  SampleTime=0
  Switch : fl_lib/Electrical/Electrical Elements/Switch  R_closed=0.01 Ohm  G_open=1e-8 1/Ohm  Threshold=0.5  i_specify=off  i_priority=None  i=0 A  i_nominal_specify=off  i_nominal_value=1  i_nominal_unit=A  v_specify=off  v_priority=None  v=0 V  v_nominal_specify=off  v_nominal_value=1  v_nominal_unit=V
  Switch1 : fl_lib/Electrical/Electrical Elements/Switch  R_closed=0.01 Ohm  G_open=1e-8 1/Ohm  Threshold=0.5  i_specify=off  i_priority=None  i=0 A  i_nominal_specify=off  i_nominal_value=1  i_nominal_unit=A  v_specify=off  v_priority=None  v=0 V  v_nominal_specify=off  v_nominal_value=1  v_nominal_unit=V
  Two-Winding Transformer (Three-Phase) : ee_lib/Passive/Transformers/Two-Winding Transformer (Three-Phase)  SRated=3.4e6 A*V  FRated=60 Hz  Winding1Connection=ee.enum.windingconnection.Yg  VRated1=13800 V  Winding2Connection=ee.enum.windingconnection.delta1  VRated2=1221 V  CoreType=ee.enum.coretype.fivelimb  pu_Rw1=0.001  pu_Rw2=0.001  leakage_reactance_option=ee.enum.transformer_leakage.include  pu_Xl1=0.03  pu_Xl2=0.03  magnetizing_resistance_option=ee.enum.transformer_magnetizingResistance.include  pu_Rm=500  magnetizing_reactance_option=ee.enum.transformer_magnetizingReactance.include  saturation_option=ee.enum.transformer_saturation.exclude  pu_Xm=500  current_data=[0, .002, 1, 2]  magnetic_flux_data=[0, 1.2, 1.5, 1.51]  pu_X0=0.5  i1_specify=on  i1_priority=High  i1=[0, 0, 0] A  i1_nominal_specify=off  i1_nominal_value=1  i1_nominal_unit=A  i2_specify=on  i2_priority=High  i2=[0, 0, 0] A  i2_nominal_specify=off  i2_nominal_value=1  i2_nominal_unit=A  phi_specify=off  phi_priority=None  phi=[0, 0, 0]  phi_nominal_specify=off  phi_nominal_value=1  phi_nominal_unit=1  power_dissipated_specify=off  power_dissipated_priority=None  power_dissipated=0 W  power_dissipated_nominal_specify=off  power_dissipated_nominal_value=1  power_dissipated_nominal_unit=W
      settings: InternalSimscapePortConfiguration="{\"Bottom\":[],\"Left\":[{\"id\":\"N1\",\"label\":\"~1\",\"type\":\"foundation.electrical.three_phase\"}],\"Right\":[{\"id\":\"N2\",\"label\":\"~2\",\"type\":\"foundation.electrical.three_phase\"}],\"Top\":[]}"
  Two-Winding Transformer (Three-Phase)1 : ee_lib/Passive/Transformers/Two-Winding Transformer (Three-Phase)  SRated=390e6 A*V  FRated=60 Hz  Winding1Connection=ee.enum.windingconnection.delta1  VRated1=13800 V  Winding2Connection=ee.enum.windingconnection.Yg  VRated2=735e3 V  CoreType=ee.enum.coretype.fivelimb  pu_Rw1=0.001  pu_Rw2=0.001  leakage_reactance_option=ee.enum.transformer_leakage.include  pu_Xl1=0.149  pu_Xl2=0.0001  magnetizing_resistance_option=ee.enum.transformer_magnetizingResistance.include  pu_Rm=500  magnetizing_reactance_option=ee.enum.transformer_magnetizingReactance.include  saturation_option=ee.enum.transformer_saturation.exclude  pu_Xm=500  current_data=[0, .002, 1, 2]  magnetic_flux_data=[0, 1.2, 1.5, 1.51]  pu_X0=0.5  i1_specify=on  i1_priority=High  i1=[0, 0, 0] A  i1_nominal_specify=off  i1_nominal_value=1  i1_nominal_unit=A  i2_specify=on  i2_priority=High  i2=[0, 0, 0] A  i2_nominal_specify=off  i2_nominal_value=1  i2_nominal_unit=A  phi_specify=off  phi_priority=None  phi=[0, 0, 0]  phi_nominal_specify=off  phi_nominal_value=1  phi_nominal_unit=1  power_dissipated_specify=off  power_dissipated_priority=None  power_dissipated=0 W  power_dissipated_nominal_specify=off  power_dissipated_nominal_value=1  power_dissipated_nominal_unit=W
      settings: InternalSimscapePortConfiguration="{\"Bottom\":[],\"Left\":[{\"id\":\"N1\",\"label\":\"~1\",\"type\":\"foundation.electrical.three_phase\"}],\"Right\":[{\"id\":\"N2\",\"label\":\"~2\",\"type\":\"foundation.electrical.three_phase\"}],\"Top\":[]}"
  Unit Delay2 : UnitDelay  InitialCondition=[1 0 0 1 0 0]  SampleTime=Ts  HasFrameUpgradeWarning=on
  VI meas : Subsystem  mask(SimScape Three-Phase VI Measurement){VoltageMeasurement=phase-to-ground, SetLabelV=on, LabelV=VabcB13_8, Vpu=on, VpuLL=off, CurrentMeasurement=yes, SetLabelI=on, LabelI=IabcB13_8, Ipu=on, Pbase=202e6, Vbase=13.8e3}
      mask prompts: VoltageMeasurement "Voltage measurement"; SetLabelV "Use a label"; LabelV "Signal label  (use a From block to collect this signal)"; Vpu "Voltages in pu,  based on peak value of nominal phase-to-ground voltage"; VpuLL "Voltages in pu,  based on peak value of nominal phase-to-phase  voltage"; CurrentMeasurement "Current measurement"; SetLabelI "Use a label"; LabelI "Signal label  (use a From block to collect this signal)"; Ipu "Currents in pu"; Pbase "Base power ( VA 3 phase)"; Vbase "Nominal voltage used for pu measurement (Vrms phase-phase) :"
      mask help:
      | Three-phase voltage and current measurements.
      |
      | The block can output the voltages and currents in per unit values or in volts and amperes.
      mask init:
      | block = gcb;
      | Kv=1;
      | Ki=1;
      | 
      | [Kv ,Ki ]=MATE3phVIMeasurementParams(block ,Vpu ,VpuLL ,Ipu ,Vbase ,Pbase);
      | MATE3phVIMeasurementCb(block ,block);
      | 
      | 
      | vtype=get_param(block,'VoltageMeasurement');
      | if isequal(vtype,'phase-to-phase')
      |     str='ee.enum.vmeasurement.ll';
      | else
      |     str= 'ee.enum.vmeasurement.lg';
      | end
      | set_param([block '/Meas'],'vMeasurementType',str);
      mask TypeOptions VoltageMeasurement: no | phase-to-ground | phase-to-phase
      mask TypeOptions CurrentMeasurement: no | yes
      mask Display: disp(['V' 10 'I']);
  VI meas1 : Subsystem  mask(SimScape Three-Phase VI Measurement){VoltageMeasurement=phase-to-ground, SetLabelV=on, LabelV=Vfault, Vpu=off, VpuLL=off, CurrentMeasurement=yes, SetLabelI=on, LabelI=Ifault, Ipu=off, Pbase=202e6, Vbase=13.8e3}
      mask prompts: VoltageMeasurement "Voltage measurement"; SetLabelV "Use a label"; LabelV "Signal label  (use a From block to collect this signal)"; Vpu "Voltages in pu,  based on peak value of nominal phase-to-ground voltage"; VpuLL "Voltages in pu,  based on peak value of nominal phase-to-phase  voltage"; CurrentMeasurement "Current measurement"; SetLabelI "Use a label"; LabelI "Signal label  (use a From block to collect this signal)"; Ipu "Currents in pu"; Pbase "Base power ( VA 3 phase)"; Vbase "Nominal voltage used for pu measurement (Vrms phase-phase) :"
      mask help:
      | Three-phase voltage and current measurements.
      |
      | The block can output the voltages and currents in per unit values or in volts and amperes.
      mask init: same as MATE_SynchronousMachine/VI meas
      mask TypeOptions VoltageMeasurement: no | phase-to-ground | phase-to-phase
      mask TypeOptions CurrentMeasurement: no | yes
      mask Display: disp(['V' 10 'I']);
  Voltage Source (Three-Phase) : ee_lib/Sources/Voltage Source (Three-Phase)  vline_rms=735e3 V  shift=0 deg  freq=60 Hz  impedance_option=1  SShortCircuit=10000e6 A*V  XR=15  R=0.01 Ohm  L=3.97e-4 H  harmonic_option=0  harmonic_orders=[5, 7, 11, 13]  harmonic_ratios=[.1, .1, .1, .1]  G_parasitic=0 1/Ohm  I_specify=on  I_priority=High  I=[0, 0, 0] A  I_nominal_specify=off  I_nominal_value=1  I_nominal_unit=A
  Voltage Sensor1 : fl_lib/Electrical/Electrical Sensors/Voltage Sensor
  Voltage Sensor2 : fl_lib/Electrical/Electrical Sensors/Voltage Sensor
  Vref : Constant
  fixed speed test1 : Constant  Value=60/20*(2*pi)
  turbine1 : Subsystem
  tag scope: I_Field=global, I_RnonLin=global, I_Sw_Field=global, I_abc=global, If=global, Pulses=global, Ucc=global, fieldON=global
  wires:
  [VabcB13_8] -> Machine and grid/1  "Vabc_B13.8 (pu)"
  [IabcB13_8] -> Math Function/1  "Iabc_B13.8"
  [I_Field] -> Machine and grid/3  "I_SwField (A)"
  [I_Field] -> Mux/1  "If (A)"
  [I_RnonLin] -> Mux/2
  [w_mec] -> Gain2/1
  [Ifault] -> Machine and grid/6  "Iabc_defaut"
  [IabcB13_8] -> -1/1
  [VabcB13_8] -> PQ/1(Vabc)
  PQ/1(PQ) -> Machine and grid/5  "P Q (pu)"
  Vref/1 -> Command/4(Vref (pu))
  [alpha] -> Machine and grid/8  "alpha (deg)"
  Gain2/1 -> Machine and grid/7  "w (pu)"
  ->pu Ifield nominal/1 -> [If], Command/3(If (pu))
  -1/1 -> PQ/2(Iabc)
  Step/1 -> [fieldON]
  Command/1(Pulses) -> Product/1
  Product/1 -> [Pulses]
  [VabcB13_8] -> Command/1(VabcB_reg (pu)), Command/2(Vabc_sync (pu))
  [I_Field] -> ->pu Ifield nominal/1
  [fieldON] -> Product/2
  Mesure et visualisation/1(V1 Vref) -> Exciter/1  "V1 - Vref (pu)"
  Mesure et visualisation/2(If IIfref) -> Exciter/2  "If - Ifref (pu)"
  Mesure et visualisation/3(Vcc) -> Exciter/3  "Vcc  - Vcc moyen (pu)"
  -2/1 -> Mux1/1
  [I_abc] -> ->pu/1  "Iabc_SM stator only"
  Mux1/1 -> Machine and grid/2  "Iabc B13.8 and SM stator (pu)"
  Mux/1 -> Machine and grid/4  "If IRnonlin (A)"
  ->pu/1 -> Mux1/2
  [fieldON] -> Simulink-PS Converter/1
  Step2/1 -> Simulink-PS Converter1/1
  MATE Synchronous Machine (p=20)/1("meas   ") -> Bus Selector2/1
  Bus Selector2/2 -> [I_Field]  "<Ifield(A)>"
  Memory2/1 -> MATE Synchronous Machine (p=20)/2("   Vfld")
  PS-Simulink Converter2/1 -> Memory2/1
  Step3/1 -> Simulink-PS Converter2/1
  Bus Selector2/1 -> [I_abc]  "<Iabc (A)>"
  Bus Selector2/3 -> [Peo]  "<Peo (W)>"
  Bus Selector2/4 -> [Te]  "<Te (Nm)>"
  [Pulses] -> Unit Delay2/1
  PS-Simulink Converter/1 -> [I_Sw_Field]
  PS-Simulink Converter1/1 -> [I_RnonLin]
  [Te] -> turbine1/2(Te)
  [fieldON] -> turbine1/1(feild)
  Manual Switch2/1 -> MATE Synchronous Machine (p=20)/1("   w_mec"), [w_mec]
  fixed speed test1/1 -> Manual Switch2/2
  [Peo] -> turbine1/3(Peo)
  turbine1/1(w) -> Manual Switch2/1
  Math Function/1 -> -2/1
  PS-Simulink Converter3/1 -> [Ucc]
  [I_Field] -> Simulink-PS Converter3/1
  Unit Delay2/1 -> MATE_LineCommutatedConverter/1(g)
  Repeating Sequence/1 -> Simulink-PS Converter4/1
  connections:
  Switch/RConn2 -- MATE_LineCommutatedConverter/RConn1 -- Voltage Sensor2/LConn1 -- Rmaintain1/LConn1
  Simulink-PS Converter/RConn1 -- Switch/RConn1
  Switch/LConn1 -- Current Sensor/LConn1
  Simulink-PS Converter1/RConn1 -- Switch1/RConn1
  Rmaintain/LConn1 -- Current Sensor/RConn2 -- Switch1/RConn2 -- Controlled Current Source/RConn2 -- Voltage Sensor1/LConn1
  Current Sensor/RConn1 -- PS-Simulink Converter/LConn1
  Current Sensor1/LConn1 -- Switch1/LConn1
  Electrical Reference1/LConn1 -- Controlled Current Source/LConn1 -- Voltage Sensor1/RConn2 -- Rmaintain/RConn1
  Voltage Sensor1/RConn1 -- PS-Simulink Converter2/LConn1
  Simulink-PS Converter3/RConn1 -- Controlled Current Source/RConn1
  Two-Winding Transformer (Three-Phase)1/LConn1 -- Circuit Breaker (Three-Phase)2/RConn1
  Two-Winding Transformer (Three-Phase)1/RConn1 -- Voltage Source (Three-Phase)/RConn1
  Electrical Reference/LConn1 -- Voltage Source (Three-Phase)/LConn1
  Circuit Breaker (Three-Phase)2/LConn1 -- Simulink-PS Converter2/RConn1
  Simulink-PS Converter4/RConn1 -- Circuit Breaker/LConn1
  MATE Synchronous Machine (p=20)/RConn1 -- Two-Winding Transformer (Three-Phase)/LConn1 -- VI meas/RConn1 -- VI meas1/RConn1
  Current Sensor1/RConn1 -- PS-Simulink Converter1/LConn1
  MATE_LineCommutatedConverter/RConn2 -- Electrical Reference3/LConn1
  Open1/LConn1 -- Electrical Reference4/LConn1
  Open1/RConn1 -- Phase Splitter/RConn2
  Open/RConn1 -- Phase Splitter/RConn3
  Open/LConn1 -- Electrical Reference5/LConn1
  VI meas1/LConn1 -- Phase Splitter/LConn1
  Current Sensor1/RConn2 -- Solver Configuration1/RConn1 -- Discharge Resistor/LConn1
  VI meas/LConn1 -- Circuit Breaker (Three-Phase)2/LConn2
  Electrical Reference6/LConn1 -- Voltage Sensor2/RConn2 -- Rmaintain1/RConn1
  Voltage Sensor2/RConn1 -- PS-Simulink Converter3/LConn1
  Circuit Breaker/LConn2 -- Phase Splitter/RConn1
  Circuit Breaker/RConn1 -- Electrical Reference2/LConn1
  Two-Winding Transformer (Three-Phase)/RConn1 -- MATE_LineCommutatedConverter/LConn1

== system MATE_SynchronousMachine/Command ==
  note: Excitation controller
  VabcB_reg (pu) : Inport
  Vabc_sync (pu) : Inport  Port=2
  If (pu) : Inport  Port=3
  Vref (pu) : Inport  Port=4
  Constant1 : Constant  Value=Iref_man
  Constant4 : Constant  Value=Auto
  Regulateur de courant : Subsystem
  Regulateur de tension (Mode automatique) : Subsystem
  Saturation : Saturate  UpperLimit=2.46  LowerLimit=0.33
  Switch : Switch  SaturateOnIntegerOverflow=off  InputSameDT=off
  "Synchro Generateur d'mpulsions " : Subsystem
  Pulses : Outport
  tag scope: Ifref=global, alpha=global
  wires:
  Vabc_sync (pu)/1 -> "Synchro Generateur d'mpulsions "/1(Vabc_138 (pu))
  "Synchro Generateur d'mpulsions "/1(P) -> Pulses/1
  VabcB_reg (pu)/1 -> Regulateur de tension (Mode automatique)/1(Vabc (pu))
  If (pu)/1 -> Regulateur de courant/1(If (pu))
  Constant4/1 -> Switch/2
  Constant1/1 -> Switch/3
  Regulateur de tension (Mode automatique)/1(Iref) -> Switch/1
  Switch/1 -> Saturation/1
  Saturation/1 -> [Ifref], Regulateur de courant/2(If_ref)
  Regulateur de courant/1(alpha) -> [alpha], "Synchro Generateur d'mpulsions "/2(alpha(deg))  "alpha (deg.)"
  Vref (pu)/1 -> Regulateur de tension (Mode automatique)/2(Vref)

== system MATE_SynchronousMachine/Discharge Resistor ==
  1-D Lookup Table : Lookup_n-D  NumberOfTableDimensions=1  BreakpointsForDimension1=[0 22 25 30 40 50 60 70 80 100 150 200 250 300 400 500 600 700 800 900 1000 1200]  Table="[0 22 25 30 40 50 60 70 80 100 150 200 250 300 400 500 600 700 800 900 1000 1200]./[1e-6 8.6250e-01 1.0500e+00 1.4250e+00 2.2500e+00 3.3750e+00 4.8750e+00 6.3750e+00 8.2500e+00  1.2000e+01 2.7750e+01 5.0250e+01 8.2500e+01 1.2000e+02 2.4000e+02 3.9750e+02 6.3750e+02 9.3750e+02 1.3125e+03 1.8000e+03 2.5500e+03 5.2500e+03]"  InternalRulePriority=Speed  RndMeth=Simplest
  Abs : Abs  SaturateOnIntegerOverflow=off
  Electrical Reference : fl_lib/Electrical/Electrical Elements/Electrical Reference
  Memory2 : Memory
  PS-Simulink Converter1 : nesl_utility/PS-Simulink Converter  PhysicalDomain=network_engine_domain  SubClassName=ps_output  LeftPortType=input  RightPortType=output  PseudoPeriodic=off  Frequencies=[]  VectorFormat=inherit  Unit=inherit  AffineConversion=off
  Simulink-PS Converter2 : nesl_utility/Simulink-PS Converter  PhysicalDomain=network_engine_domain  SubClassName=ps_input  LeftPortType=input  RightPortType=output  PseudoPeriodic=off  Frequencies=[]  NoiseDistribution=none  NoiseParameters=[]  Unit=1  AffineConversion=off  FilteringAndDerivatives=provide  SimscapeFilterOrder=1  InputFilterTimeConstant=0.001  UdotUserProvided=0
  Variable Resistor : fl_lib/Electrical/Electrical Elements/Variable Resistor  Rmin=0 Ohm  thermalEnable=false  thermal_mass=1 J/K  i_specify=off  i_priority=None  i=0 A  i_nominal_specify=off  i_nominal_value=1  i_nominal_unit=A  v_specify=off  v_priority=None  v=0 V  v_nominal_specify=off  v_nominal_value=1  v_nominal_unit=V  T_specify=off  T_priority=None  T=300 K  T_nominal_specify=off  T_nominal_value=1  T_nominal_unit=K
  Voltage Sensor : fl_lib/Electrical/Electrical Sensors/Voltage Sensor
  Conn1 : PMIOPort  Side=Left
  wires:
  PS-Simulink Converter1/1 -> Abs/1
  1-D Lookup Table/1 -> Memory2/1
  Memory2/1 -> Simulink-PS Converter2/1
  Abs/1 -> 1-D Lookup Table/1
  connections:
  Voltage Sensor/RConn2 -- Variable Resistor/RConn1 -- Electrical Reference/LConn1
  Voltage Sensor/RConn1 -- PS-Simulink Converter1/LConn1
  Voltage Sensor/LConn1 -- Conn1/RConn1 -- Variable Resistor/LConn2
  Simulink-PS Converter2/RConn1 -- Variable Resistor/LConn1
